simulink model "sim_5"  (R2015b)
settings: Solver=ode45  StartTime=0  StopTime=2000  FixedStep=1e-3  RelTol=1e-4
values from neighbouring files (symbols this model uses):
  alpha_nc = 5*pi/2    (= 7.85398163397)    [run_sim5.m]
  alpha_nw = 3*pi/4    (= 2.35619449019)    [run_sim5.m]
  U_mean_c = 1    [run_sim5.m]
  U_mean_w = 15    [run_sim5.m]
undefined symbols (not defined in the file or in its folder): B, currentCoeffMatrix, D, E, f, H, h, K2_np, K3_np, K4_np, Kd_surge, Kd_sway, Kd_yaw, Ki_surge, Ki_sway, Ki_yaw, Kp_surge, Kp_sway, Kp_yaw, M_inverse, mu, N_freq, P0, Par, phi, Q, R, S, Sim, T_pinv, TA_sampling_time, thrusterPositionX, thrusterPositionY, thrusters, thrustersInitialAlpha, windCoeffMatrix, x0
libraries: simulink_extras x8, marine_gnc x5, simulink x5
(part 2 of 2)

== matlab function sim_5/Env_NEW/get wind coeffcients ==
  data: alpha input; C output; windCoeffMatrix input
function C   = WindCoeffcients(alpha, windCoeffMatrix)
% Initialization of the return parameter
C=zeros(6,1);

while alpha > 360
    alpha = alpha - 360;
end

while alpha < 0
    alpha = alpha + 360;
end

alpha_mod = mod(alpha,10);
avrundet_alpha = alpha - alpha_mod;
index = avrundet_alpha/10+1;

C1 = windCoeffMatrix(index,:)';
C2 = windCoeffMatrix(index+1,:)';

for i = 1:6
    diff = C2(i)-C1(i);
    point = (diff/10)*alpha_mod;
    C(i) = C1(i)+point;
end

end
